simulink model "MATLABPSB_BASED_MODELING_AND_Sim"  (Simulink 8.1)
settings: Solver=FixedStepDiscrete  SolverMode=SingleTasking  StartTime=0.0  StopTime=1  FixedStep=Ts  MaxStep=Ts*2  RelTol=1e-4  AbsTol=1e-4
PreLoadFcn:
  | Ts=50e-6;
values from neighbouring files (symbols this model uses):
  A = 1.5    [LoadSimulation.m]
undefined symbols (not defined in the file or in its folder): DiscIntNeverNeededParam, find_system
libraries: powerlib x205, powerlib_extras x39
(part 4 of 5)

== system MATLABPSB_BASED_MODELING_AND_Sim/SS1/SVC Controller/Firing Unit/Firing Unit BC/BL8 ==
  Ns/c : Inport
  Alpha : Inport  Port=2  PortDimensions=1
  Sync + : Inport  Port=3  PortDimensions=1
  SqWave : Inport  Port=4  PortDimensions=1
  Alpha 90<A<181 : Constant  Value=90
  Alpha 90<A<182 : Constant  Value=360
  Alpha 90<A<183 : Constant  Value=2
  Alpha 90<A<184 : Constant  Value=2
  Alpha 90<A<185 : Constant  Value=87
  Discrete-Time Integrator : DiscreteIntegrator  ExternalReset=rising  SampleTime=Ts  LimitOutput=on  UpperSaturationLimit=100000  LowerSaturationLimit=0  ICPrevOutput=DiscIntNeverNeededParam  ICPrevScaledInput=DiscIntNeverNeededParam
  Gain2 : Gain  Gain=1/Ts  SaturateOnIntegerOverflow=on  OutDataTypeStr=Inherit: Same as input  ParamDataTypeStr=Inherit: Same as input
  Logical Operator1 : Logic  Inputs=3
  Logical Operator2 : Logic  Operator=NOT  Inputs=3
  Product : Product  Inputs=*/  SaturateOnIntegerOverflow=on  InputSameDT=on  OutDataTypeStr=Inherit: Same as first input
  Product1 : Product  Inputs=**  SaturateOnIntegerOverflow=on  InputSameDT=on  OutDataTypeStr=Inherit: Same as first input
  Product2 : Product  Inputs=*/  SaturateOnIntegerOverflow=on  InputSameDT=on  OutDataTypeStr=Inherit: Same as first input
  Relational Operator1 : RelationalOperator  Operator=<=  InputSameDT=on
  Relational Operator2 : RelationalOperator  InputSameDT=on
  Relational Operator3 : RelationalOperator  Operator=<=  InputSameDT=on
  Rounding Function1 : Rounding  Operator=round
  Rounding Function3 : Rounding  Operator=round
  Sum1 : Sum  Inputs=+-  SaturateOnIntegerOverflow=on  InputSameDT=on  OutDataTypeStr=Inherit: Same as first input
  Sum2 : Sum  Inputs=+--  SaturateOnIntegerOverflow=on  InputSameDT=on  OutDataTypeStr=Inherit: Same as first input
  Switch : Switch  Threshold=0.5  SaturateOnIntegerOverflow=on  InputSameDT=on
  Switch1 : Switch  Threshold=0.5  SaturateOnIntegerOverflow=on  InputSameDT=on
  Unit Delay1 : UnitDelay  InitialCondition=180  SampleTime=Ts
  TCR + : Outport
  wires:
  Switch1/1 -> Sum1/1, Unit Delay1/1
  Alpha 90<A<181/1 -> Sum1/2
  Ns/c/1 -> Product1/1, Product2/1
  Product1/1 -> Rounding Function1/1
  Alpha 90<A<182/1 -> Product/2
  Product/1 -> Product1/2
  Product2/1 -> Rounding Function3/1
  Alpha 90<A<183/1 -> Product2/2
  Sum1/1 -> Product/1, Relational Operator1/1
  Alpha 90<A<185/1 -> Relational Operator1/2
  Unit Delay1/1 -> Switch1/3
  Alpha/1 -> Switch1/1
  Rounding Function1/1 -> Sum2/3, Switch/1
  Rounding Function3/1 -> Sum2/1, Switch/3
  Alpha 90<A<184/1 -> Sum2/2
  Relational Operator1/1 -> Switch/2
  Relational Operator3/1 -> Logical Operator1/3
  Discrete-Time Integrator/1 -> Relational Operator2/1, Relational Operator3/1
  Relational Operator2/1 -> Logical Operator1/2
  Logical Operator1/1 -> TCR +/1
  Gain2/1 -> Discrete-Time Integrator/1
  Switch/1 -> Relational Operator2/2
  Sum2/1 -> Relational Operator3/2
  Logical Operator2/1 -> Discrete-Time Integrator/2
  Sync +/1 -> Switch1/2
  SqWave/1 -> Gain2/1, Logical Operator2/1, Logical Operator1/1

== system MATLABPSB_BASED_MODELING_AND_Sim/SS1/SVC Controller/Firing Unit/Firing Unit CA/BL1 ==
  note: Pierre Giroux, Gilbert Sybille
      | Power System Laboratory, IREQ
      | Hydro-Quebec
  note: Note: PLL synchronized on positive peak of input
  note: Discrete 1-phase PLL
  note: Note: -sin( a ) * sin( b ) = 1/2 * cos( a+b ) - 1/2 * cos(a-b)
  V(pu) : Inport
  Constant4 : Constant  Value=2*pi
  Discrete PI Controller : powerlib_extras/Discrete  Control Blocks/Discrete PI Controller  Kp=Kp  Ki=Ki  Par_Limits="[1.25  0.75]*2*pi*Finit"  Init=2*pi*Finit  Ts=Ts
  Discrete Rate Limiter : powerlib_extras/Discrete  Control Blocks/Discrete Rate Limiter  R=10  F=-10  Vinit=Finit  Ts=Ts
  Discrete Variable Frequency Mean value : powerlib_extras/Discrete Measurements/Discrete Variable Frequency Mean value  Finit=Finit  Fmin=45  Vinit=0  Ts=Ts
  Discrete  2nd-Order Filter : powerlib_extras/Discrete  Control Blocks/Discrete  2nd-Order Filter  FilterType=Lowpass  Fo=25  Zeta=0.707  Ts=Ts  Initialize=on  Vac_Init="[0 0  Finit]"  Vdc_Init=Finit  PlotResponse=off  param1=[1 500 0.1]
  Discrete-Time Integrator : DiscreteIntegrator  InitialCondition=(Phase_Init-90)*pi/180  SampleTime=Ts  ICPrevOutput=DiscIntNeverNeededParam  ICPrevScaledInput=DiscIntNeverNeededParam
  Gain10 : Gain  Gain=1/2/pi  SaturateOnIntegerOverflow=on  OutDataTypeStr=Inherit: Same as input  ParamDataTypeStr=Inherit: Same as input
  Gain12 : Gain  Gain=-1  SaturateOnIntegerOverflow=on  OutDataTypeStr=Inherit: Same as input  ParamDataTypeStr=Inherit: Same as input
  Math Function : Math  Operator=mod  SaturateOnIntegerOverflow=on
  Product1 : Product  SaturateOnIntegerOverflow=on  InputSameDT=on  OutDataTypeStr=Inherit: Same as first input
  Trigonometric Function6 : Trigonometry
  Unit Delay1 : UnitDelay  InitialCondition=Finit  SampleTime=Ts
  Freq : Outport
  wt : Outport  Port=2
  wires:
  Math Function/1 -> wt/1, Trigonometric Function6/1
  Trigonometric Function6/1 -> Product1/2
  Unit Delay1/1 -> Discrete Variable Frequency Mean value/1, Freq/1
  Discrete  2nd-Order Filter/1 -> Unit Delay1/1
  Discrete Rate Limiter/1 -> Discrete  2nd-Order Filter/1
  Gain10/1 -> Discrete Rate Limiter/1
  Discrete PI Controller/1 -> Gain10/1, Discrete-Time Integrator/1  "W"
  Product1/1 -> Discrete Variable Frequency Mean value/2
  Discrete Variable Frequency Mean value/1 -> Discrete PI Controller/1
  Discrete-Time Integrator/1 -> Math Function/1
  Constant4/1 -> Math Function/2
  V(pu)/1 -> Gain12/1
  Gain12/1 -> Product1/1

== system MATLABPSB_BASED_MODELING_AND_Sim/SS1/SVC Controller/Firing Unit/Firing Unit CA/BL2 ==
  Freq : Inport  PortDimensions=1
  Constant1 : Constant  Value=0
  Constant2 : Constant  Value=1e-5
  Constant3 : Constant
  Gain : Gain  Gain=Ts  SaturateOnIntegerOverflow=on  OutDataTypeStr=Inherit: Same as input  ParamDataTypeStr=Inherit: Same as input
  Product : Product  Inputs=/*  SaturateOnIntegerOverflow=on  InputSameDT=on  OutDataTypeStr=Inherit: Same as first input
  Relational Operator1 : RelationalOperator  Operator=~=  InputSameDT=on
  Switch : Switch  Threshold=0.5  SaturateOnIntegerOverflow=on  InputSameDT=on
  Ns/c : Outport
  wires:
  Constant3/1 -> Product/2
  Switch/1 -> Product/1
  Relational Operator1/1 -> Switch/2
  Constant2/1 -> Switch/3
  Gain/1 -> Switch/1, Relational Operator1/1
  Constant1/1 -> Relational Operator1/2
  Freq/1 -> Gain/1
  Product/1 -> Ns/c/1

== system MATLABPSB_BASED_MODELING_AND_Sim/SS1/SVC Controller/Firing Unit/Firing Unit CA/BL3 ==
  Freq : Inport  PortDimensions=1
  sin(wt) : Inport  Port=2  PortDimensions=1
  Latch : Subsystem
  Logical Operator2 : Logic
  Logical Operator4 : Logic
  Product2 : Product  SaturateOnIntegerOverflow=on  InputSameDT=on  OutDataTypeStr=Inherit: Same as first input
  Relational Operator : RelationalOperator  Operator=>  InputSameDT=on
  Relational Operator1 : RelationalOperator  Operator=>  InputSameDT=on
  Relational Operator2 : RelationalOperator  Operator=<  InputSameDT=on
  Relational Operator3 : RelationalOperator  Operator=<  InputSameDT=on
  Scope : Scope
      settings: YMin=-0.0004  YMax=0.0004  SampleInput=on  SampleTime=Ts
  Sum5 : Sum  Inputs=+-  SaturateOnIntegerOverflow=on  InputSameDT=on  OutDataTypeStr=Inherit: Same as first input
  Sum6 : Sum  SaturateOnIntegerOverflow=on  InputSameDT=on  OutDataTypeStr=Inherit: Same as first input
  Trigonometric Function7 : Trigonometry
  Unit Delay : UnitDelay  SampleTime=Ts
  Unit Delay1 : UnitDelay  SampleTime=Ts
  Unit Delay2 : UnitDelay  SampleTime=Ts
  alpha2 : Constant  Value=0
  alpha9 : Constant  Value=pi*Ts
  SqWave : Outport
  Sync + : Outport  Port=2
  Sync - : Outport  Port=3
  wires:
  alpha9/1 -> Product2/1
  Product2/1 -> Trigonometric Function7/1
  Latch/1(1) -> SqWave/1, Unit Delay1/1, Unit Delay2/1, Relational Operator1/1, Relational Operator3/1
  Unit Delay1/1 -> Logical Operator4/2
  Logical Operator4/1 -> Latch/2(R)
  Relational Operator2/1 -> Logical Operator4/1
  Unit Delay/1 -> Logical Operator2/2
  Latch/2(0) -> Unit Delay/1
  Logical Operator2/1 -> Latch/1(S)
  Relational Operator/1 -> Logical Operator2/1
  Sum6/1 -> Relational Operator2/2
  Sum5/1 -> Relational Operator/2
  alpha2/1 -> Sum6/1, Sum5/1
  Relational Operator1/1 -> Sync +/1
  Relational Operator3/1 -> Sync -/1
  Unit Delay2/1 -> Relational Operator1/2, Relational Operator3/2
  Trigonometric Function7/1 -> Sum6/2, Sum5/2, Scope/1
  Freq/1 -> Product2/2
  sin(wt)/1 -> Relational Operator/1, Relational Operator2/1

== system MATLABPSB_BASED_MODELING_AND_Sim/SS1/SVC Controller/Firing Unit/Firing Unit CA/BL4 ==
  note: Note: Sync+ , Sync - and SqWave signals are inverted for TSC firing (i.e. positive thyristor is fired on negative peak voltage)
  SqWave : Inport  PortDimensions=1
  Sync + : Inport  Port=2  PortDimensions=1
  Sync - : Inport  Port=3  PortDimensions=1
  TSC_On : Inport  Port=4  PortDimensions=1
  Alpha1 : Constant  Value=FiringMode-1
  Logical Operator1 : Logic  Operator=NOT
  Logical Operator10 : Logic  Operator=OR
  Logical Operator11 : Logic  Inputs=3
  Logical Operator12 : Logic
  Logical Operator13 : Logic
  Logical Operator14 : Logic  Operator=OR
  Logical Operator15 : Logic  Inputs=3
  Switch5 : Switch  Threshold=0.5  SaturateOnIntegerOverflow=on  InputSameDT=on
  Switch6 : Switch  Threshold=0.5  SaturateOnIntegerOverflow=on  InputSameDT=on
  Transport Delay : TransportDelay  DelayTime=1/FreqInit  BufferSize=2048
  Unit Delay6 : UnitDelay  SampleTime=Ts
  Unit Delay7 : UnitDelay  SampleTime=Ts
  TSC + : Outport
  TSC - : Outport  Port=2
  wires:
  Transport Delay/1 -> Logical Operator14/2, Logical Operator10/2
  Logical Operator15/1 -> TSC -/1
  Logical Operator11/1 -> TSC +/1
  Logical Operator14/1 -> Logical Operator15/2
  Logical Operator10/1 -> Logical Operator11/2
  Logical Operator1/1 -> Logical Operator10/1
  Switch6/1 -> Logical Operator15/1, Logical Operator13/2, Unit Delay7/1
  Switch5/1 -> Logical Operator11/1, Logical Operator13/1, Unit Delay6/1
  SqWave/1 -> Logical Operator14/1, Logical Operator1/1
  Logical Operator12/1 -> Transport Delay/1
  Alpha1/1 -> Logical Operator12/2
  Logical Operator13/1 -> Logical Operator12/1
  TSC_On/1 -> Logical Operator15/3, Logical Operator11/3, Switch6/1, Switch5/1
  Sync -/1 -> Switch5/2
  Sync +/1 -> Switch6/2
  Unit Delay7/1 -> Switch6/3
  Unit Delay6/1 -> Switch5/3

== system MATLABPSB_BASED_MODELING_AND_Sim/SS1/SVC Controller/Firing Unit/Firing Unit CA/BL5 ==
  note: Note: Sync+ , Sync - and SqWave signals are inverted for TSC firing (i.e. positive thyristor is fired on negative peak voltage)
  SqWave : Inport  PortDimensions=1
  Sync + : Inport  Port=2  PortDimensions=1
  Sync - : Inport  Port=3  PortDimensions=1
  TSC_On : Inport  Port=4  PortDimensions=1
  Alpha1 : Constant  Value=FiringMode-1
  Logical Operator1 : Logic  Operator=NOT
  Logical Operator10 : Logic  Operator=OR
  Logical Operator11 : Logic  Inputs=3
  Logical Operator12 : Logic
  Logical Operator13 : Logic
  Logical Operator14 : Logic  Operator=OR
  Logical Operator15 : Logic  Inputs=3
  Switch5 : Switch  Threshold=0.5  SaturateOnIntegerOverflow=on  InputSameDT=on
  Switch6 : Switch  Threshold=0.5  SaturateOnIntegerOverflow=on  InputSameDT=on
  Transport Delay : TransportDelay  DelayTime=1/FreqInit  BufferSize=2048
  Unit Delay6 : UnitDelay  SampleTime=Ts
  Unit Delay7 : UnitDelay  SampleTime=Ts
  TSC + : Outport
  TSC - : Outport  Port=2
  wires:
  Unit Delay6/1 -> Switch5/3
  Unit Delay7/1 -> Switch6/3
  Sync +/1 -> Switch6/2
  Sync -/1 -> Switch5/2
  TSC_On/1 -> Switch5/1, Switch6/1, Logical Operator11/3, Logical Operator15/3
  Logical Operator13/1 -> Logical Operator12/1
  Alpha1/1 -> Logical Operator12/2
  Logical Operator12/1 -> Transport Delay/1
  SqWave/1 -> Logical Operator1/1, Logical Operator14/1
  Switch5/1 -> Unit Delay6/1, Logical Operator13/1, Logical Operator11/1
  Switch6/1 -> Unit Delay7/1, Logical Operator13/2, Logical Operator15/1
  Logical Operator1/1 -> Logical Operator10/1
  Logical Operator10/1 -> Logical Operator11/2
  Logical Operator14/1 -> Logical Operator15/2
  Logical Operator11/1 -> TSC +/1
  Logical Operator15/1 -> TSC -/1
  Transport Delay/1 -> Logical Operator10/2, Logical Operator14/2

== system MATLABPSB_BASED_MODELING_AND_Sim/SS1/SVC Controller/Firing Unit/Firing Unit CA/BL6 ==
  note: Note: Sync+ , Sync - and SqWave signals are inverted for TSC firing (i.e. positive thyristor is fired on negative peak voltage)
  SqWave : Inport  PortDimensions=1
  Sync + : Inport  Port=2  PortDimensions=1
  Sync - : Inport  Port=3  PortDimensions=1
  TSC_On : Inport  Port=4  PortDimensions=1
  Alpha1 : Constant  Value=FiringMode-1
  Logical Operator1 : Logic  Operator=NOT
  Logical Operator10 : Logic  Operator=OR
  Logical Operator11 : Logic  Inputs=3
  Logical Operator12 : Logic
  Logical Operator13 : Logic
  Logical Operator14 : Logic  Operator=OR
  Logical Operator15 : Logic  Inputs=3
  Switch5 : Switch  Threshold=0.5  SaturateOnIntegerOverflow=on  InputSameDT=on
  Switch6 : Switch  Threshold=0.5  SaturateOnIntegerOverflow=on  InputSameDT=on
  Transport Delay : TransportDelay  DelayTime=1/FreqInit  BufferSize=2048
  Unit Delay6 : UnitDelay  SampleTime=Ts
  Unit Delay7 : UnitDelay  SampleTime=Ts
  TSC + : Outport
  TSC - : Outport  Port=2
  wires:
  Transport Delay/1 -> Logical Operator14/2, Logical Operator10/2
  Logical Operator15/1 -> TSC -/1
  Logical Operator11/1 -> TSC +/1
  Logical Operator14/1 -> Logical Operator15/2
  Logical Operator10/1 -> Logical Operator11/2
  Logical Operator1/1 -> Logical Operator10/1
  Switch6/1 -> Logical Operator15/1, Logical Operator13/2, Unit Delay7/1
  Switch5/1 -> Logical Operator11/1, Logical Operator13/1, Unit Delay6/1
  SqWave/1 -> Logical Operator14/1, Logical Operator1/1
  Logical Operator12/1 -> Transport Delay/1
  Alpha1/1 -> Logical Operator12/2
  Logical Operator13/1 -> Logical Operator12/1
  TSC_On/1 -> Logical Operator15/3, Logical Operator11/3, Switch6/1, Switch5/1
  Sync -/1 -> Switch5/2
  Sync +/1 -> Switch6/2
  Unit Delay7/1 -> Switch6/3
  Unit Delay6/1 -> Switch5/3

== system MATLABPSB_BASED_MODELING_AND_Sim/SS1/SVC Controller/Firing Unit/Firing Unit CA/BL7 ==
  Ns/c : Inport
  Alpha : Inport  Port=2  PortDimensions=1
  Sync - : Inport  Port=3  PortDimensions=1
  SqWave : Inport  Port=4  PortDimensions=1
  Alpha 90<A<181 : Constant  Value=90
  Alpha 90<A<182 : Constant  Value=360
  Alpha 90<A<183 : Constant  Value=2
  Alpha 90<A<184 : Constant  Value=2
  Alpha 90<A<185 : Constant  Value=87
  Discrete-Time Integrator : DiscreteIntegrator  ExternalReset=rising  SampleTime=Ts  LimitOutput=on  UpperSaturationLimit=100000  LowerSaturationLimit=0  ICPrevOutput=DiscIntNeverNeededParam  ICPrevScaledInput=DiscIntNeverNeededParam
  Gain2 : Gain  Gain=1/Ts  SaturateOnIntegerOverflow=on  OutDataTypeStr=Inherit: Same as input  ParamDataTypeStr=Inherit: Same as input
  Logical Operator1 : Logic  Inputs=3
  Logical Operator2 : Logic  Operator=NOT  Inputs=3
  Logical Operator3 : Logic  Operator=NOT  Inputs=3
  Product : Product  Inputs=*/  SaturateOnIntegerOverflow=on  InputSameDT=on  OutDataTypeStr=Inherit: Same as first input
  Product1 : Product  Inputs=**  SaturateOnIntegerOverflow=on  InputSameDT=on  OutDataTypeStr=Inherit: Same as first input
  Product2 : Product  Inputs=*/  SaturateOnIntegerOverflow=on  InputSameDT=on  OutDataTypeStr=Inherit: Same as first input
  Relational Operator1 : RelationalOperator  Operator=<=  InputSameDT=on
  Relational Operator2 : RelationalOperator  InputSameDT=on
  Relational Operator3 : RelationalOperator  Operator=<=  InputSameDT=on
  Rounding Function1 : Rounding  Operator=round
  Rounding Function3 : Rounding  Operator=round
  Sum1 : Sum  Inputs=+-  SaturateOnIntegerOverflow=on  InputSameDT=on  OutDataTypeStr=Inherit: Same as first input
  Sum2 : Sum  Inputs=+--  SaturateOnIntegerOverflow=on  InputSameDT=on  OutDataTypeStr=Inherit: Same as first input
  Switch : Switch  Threshold=0.5  SaturateOnIntegerOverflow=on  InputSameDT=on
  Switch1 : Switch  Threshold=0.5  SaturateOnIntegerOverflow=on  InputSameDT=on
  Unit Delay1 : UnitDelay  InitialCondition=180  SampleTime=Ts
  TCR - : Outport
  wires:
  Switch1/1 -> Sum1/1, Unit Delay1/1
  Alpha 90<A<181/1 -> Sum1/2
  Ns/c/1 -> Product1/1, Product2/1
  Product1/1 -> Rounding Function1/1
  Alpha 90<A<182/1 -> Product/2
  Product/1 -> Product1/2
  Product2/1 -> Rounding Function3/1
  Alpha 90<A<183/1 -> Product2/2
  Sum1/1 -> Product/1, Relational Operator1/1
  Alpha 90<A<185/1 -> Relational Operator1/2
  Unit Delay1/1 -> Switch1/3
  Alpha/1 -> Switch1/1
  Rounding Function1/1 -> Sum2/3, Switch/1
  Rounding Function3/1 -> Sum2/1, Switch/3
  Alpha 90<A<184/1 -> Sum2/2
  Relational Operator1/1 -> Switch/2
  Relational Operator3/1 -> Logical Operator1/3
  Discrete-Time Integrator/1 -> Relational Operator2/1, Relational Operator3/1
  Relational Operator2/1 -> Logical Operator1/2
  Logical Operator1/1 -> TCR -/1
  Gain2/1 -> Discrete-Time Integrator/1
  Switch/1 -> Relational Operator2/2
  Sum2/1 -> Relational Operator3/2
  Logical Operator2/1 -> Discrete-Time Integrator/2
  Sync -/1 -> Switch1/2
  SqWave/1 -> Logical Operator3/1
  Logical Operator3/1 -> Gain2/1, Logical Operator2/1, Logical Operator1/1

== system MATLABPSB_BASED_MODELING_AND_Sim/SS1/SVC Controller/Firing Unit/Firing Unit CA/BL8 ==
  Ns/c : Inport
  Alpha : Inport  Port=2  PortDimensions=1
  Sync + : Inport  Port=3  PortDimensions=1
  SqWave : Inport  Port=4  PortDimensions=1
  Alpha 90<A<181 : Constant  Value=90
  Alpha 90<A<182 : Constant  Value=360
  Alpha 90<A<183 : Constant  Value=2
  Alpha 90<A<184 : Constant  Value=2
  Alpha 90<A<185 : Constant  Value=87
  Discrete-Time Integrator : DiscreteIntegrator  ExternalReset=rising  SampleTime=Ts  LimitOutput=on  UpperSaturationLimit=100000  LowerSaturationLimit=0  ICPrevOutput=DiscIntNeverNeededParam  ICPrevScaledInput=DiscIntNeverNeededParam
  Gain2 : Gain  Gain=1/Ts  SaturateOnIntegerOverflow=on  OutDataTypeStr=Inherit: Same as input  ParamDataTypeStr=Inherit: Same as input
  Logical Operator1 : Logic  Inputs=3
  Logical Operator2 : Logic  Operator=NOT  Inputs=3
  Product : Product  Inputs=*/  SaturateOnIntegerOverflow=on  InputSameDT=on  OutDataTypeStr=Inherit: Same as first input
  Product1 : Product  Inputs=**  SaturateOnIntegerOverflow=on  InputSameDT=on  OutDataTypeStr=Inherit: Same as first input
  Product2 : Product  Inputs=*/  SaturateOnIntegerOverflow=on  InputSameDT=on  OutDataTypeStr=Inherit: Same as first input
  Relational Operator1 : RelationalOperator  Operator=<=  InputSameDT=on
  Relational Operator2 : RelationalOperator  InputSameDT=on
  Relational Operator3 : RelationalOperator  Operator=<=  InputSameDT=on
  Rounding Function1 : Rounding  Operator=round
  Rounding Function3 : Rounding  Operator=round
  Sum1 : Sum  Inputs=+-  SaturateOnIntegerOverflow=on  InputSameDT=on  OutDataTypeStr=Inherit: Same as first input
  Sum2 : Sum  Inputs=+--  SaturateOnIntegerOverflow=on  InputSameDT=on  OutDataTypeStr=Inherit: Same as first input
  Switch : Switch  Threshold=0.5  SaturateOnIntegerOverflow=on  InputSameDT=on
  Switch1 : Switch  Threshold=0.5  SaturateOnIntegerOverflow=on  InputSameDT=on
  Unit Delay1 : UnitDelay  InitialCondition=180  SampleTime=Ts
  TCR + : Outport
  wires:
  SqWave/1 -> Logical Operator1/1, Logical Operator2/1, Gain2/1
  Sync +/1 -> Switch1/2
  Logical Operator2/1 -> Discrete-Time Integrator/2
  Sum2/1 -> Relational Operator3/2
  Switch/1 -> Relational Operator2/2
  Gain2/1 -> Discrete-Time Integrator/1
  Logical Operator1/1 -> TCR +/1
  Relational Operator2/1 -> Logical Operator1/2
  Discrete-Time Integrator/1 -> Relational Operator3/1, Relational Operator2/1
  Relational Operator3/1 -> Logical Operator1/3
  Relational Operator1/1 -> Switch/2
  Alpha 90<A<184/1 -> Sum2/2
  Rounding Function3/1 -> Switch/3, Sum2/1
  Rounding Function1/1 -> Switch/1, Sum2/3
  Alpha/1 -> Switch1/1
  Unit Delay1/1 -> Switch1/3
  Alpha 90<A<185/1 -> Relational Operator1/2
  Sum1/1 -> Relational Operator1/1, Product/1
  Alpha 90<A<183/1 -> Product2/2
  Product2/1 -> Rounding Function3/1
  Product/1 -> Product1/2
  Alpha 90<A<182/1 -> Product/2
  Product1/1 -> Rounding Function1/1
  Ns/c/1 -> Product2/1, Product1/1
  Alpha 90<A<181/1 -> Sum1/2
  Switch1/1 -> Unit Delay1/1, Sum1/1

== system MATLABPSB_BASED_MODELING_AND_Sim/SS2/SVC Controller/Firing Unit/Firing Unit AB/BL1 ==
  note: Pierre Giroux, Gilbert Sybille
      | Power System Laboratory, IREQ
      | Hydro-Quebec
  note: Note: PLL synchronized on positive peak of input
  note: Discrete 1-phase PLL
  note: Note: -sin( a ) * sin( b ) = 1/2 * cos( a+b ) - 1/2 * cos(a-b)
  V(pu) : Inport
  Constant4 : Constant  Value=2*pi
  Discrete PI Controller : powerlib_extras/Discrete  Control Blocks/Discrete PI Controller  Kp=Kp  Ki=Ki  Par_Limits="[1.25  0.75]*2*pi*Finit"  Init=2*pi*Finit  Ts=Ts
  Discrete Rate Limiter : powerlib_extras/Discrete  Control Blocks/Discrete Rate Limiter  R=10  F=-10  Vinit=Finit  Ts=Ts
  Discrete Variable Frequency Mean value : powerlib_extras/Discrete Measurements/Discrete Variable Frequency Mean value  Finit=Finit  Fmin=45  Vinit=0  Ts=Ts
  Discrete  2nd-Order Filter : powerlib_extras/Discrete  Control Blocks/Discrete  2nd-Order Filter  FilterType=Lowpass  Fo=25  Zeta=0.707  Ts=Ts  Initialize=on  Vac_Init="[0 0  Finit]"  Vdc_Init=Finit  PlotResponse=off  param1=[1 500 0.1]
  Discrete-Time Integrator : DiscreteIntegrator  InitialCondition=(Phase_Init-90)*pi/180  SampleTime=Ts  ICPrevOutput=DiscIntNeverNeededParam  ICPrevScaledInput=DiscIntNeverNeededParam
  Gain10 : Gain  Gain=1/2/pi  SaturateOnIntegerOverflow=on  OutDataTypeStr=Inherit: Same as input  ParamDataTypeStr=Inherit: Same as input
  Gain12 : Gain  Gain=-1  SaturateOnIntegerOverflow=on  OutDataTypeStr=Inherit: Same as input  ParamDataTypeStr=Inherit: Same as input
  Math Function : Math  Operator=mod  SaturateOnIntegerOverflow=on
  Product1 : Product  SaturateOnIntegerOverflow=on  InputSameDT=on  OutDataTypeStr=Inherit: Same as first input
  Trigonometric Function6 : Trigonometry
  Unit Delay1 : UnitDelay  InitialCondition=Finit  SampleTime=Ts
  Freq : Outport
  wt : Outport  Port=2
  wires:
  Math Function/1 -> wt/1, Trigonometric Function6/1
  Trigonometric Function6/1 -> Product1/2
  Unit Delay1/1 -> Discrete Variable Frequency Mean value/1, Freq/1
  Discrete  2nd-Order Filter/1 -> Unit Delay1/1
  Discrete Rate Limiter/1 -> Discrete  2nd-Order Filter/1
  Gain10/1 -> Discrete Rate Limiter/1
  Discrete PI Controller/1 -> Gain10/1, Discrete-Time Integrator/1  "W"
  Product1/1 -> Discrete Variable Frequency Mean value/2
  Discrete Variable Frequency Mean value/1 -> Discrete PI Controller/1
  Discrete-Time Integrator/1 -> Math Function/1
  Constant4/1 -> Math Function/2
  V(pu)/1 -> Gain12/1
  Gain12/1 -> Product1/1

== system MATLABPSB_BASED_MODELING_AND_Sim/SS2/SVC Controller/Firing Unit/Firing Unit AB/BL2 ==
  Freq : Inport  PortDimensions=1
  Constant1 : Constant  Value=0
  Constant2 : Constant  Value=1e-5
  Constant3 : Constant
  Gain : Gain  Gain=Ts  SaturateOnIntegerOverflow=on  OutDataTypeStr=Inherit: Same as input  ParamDataTypeStr=Inherit: Same as input
  Product : Product  Inputs=/*  SaturateOnIntegerOverflow=on  InputSameDT=on  OutDataTypeStr=Inherit: Same as first input
  Relational Operator1 : RelationalOperator  Operator=~=  InputSameDT=on
  Switch : Switch  Threshold=0.5  SaturateOnIntegerOverflow=on  InputSameDT=on
  Ns/c : Outport
  wires:
  Constant3/1 -> Product/2
  Switch/1 -> Product/1
  Relational Operator1/1 -> Switch/2
  Constant2/1 -> Switch/3
  Gain/1 -> Switch/1, Relational Operator1/1
  Constant1/1 -> Relational Operator1/2
  Freq/1 -> Gain/1
  Product/1 -> Ns/c/1

== system MATLABPSB_BASED_MODELING_AND_Sim/SS2/SVC Controller/Firing Unit/Firing Unit AB/BL3 ==
  Freq : Inport  PortDimensions=1
  sin(wt) : Inport  Port=2  PortDimensions=1
  Latch : Subsystem
  Logical Operator2 : Logic
  Logical Operator4 : Logic
  Product2 : Product  SaturateOnIntegerOverflow=on  InputSameDT=on  OutDataTypeStr=Inherit: Same as first input
  Relational Operator : RelationalOperator  Operator=>  InputSameDT=on
  Relational Operator1 : RelationalOperator  Operator=>  InputSameDT=on
  Relational Operator2 : RelationalOperator  Operator=<  InputSameDT=on
  Relational Operator3 : RelationalOperator  Operator=<  InputSameDT=on
  Scope : Scope
      settings: YMin=-0.0004  YMax=0.0004  SampleInput=on  SampleTime=Ts
  Sum5 : Sum  Inputs=+-  SaturateOnIntegerOverflow=on  InputSameDT=on  OutDataTypeStr=Inherit: Same as first input
  Sum6 : Sum  SaturateOnIntegerOverflow=on  InputSameDT=on  OutDataTypeStr=Inherit: Same as first input
  Trigonometric Function7 : Trigonometry
  Unit Delay : UnitDelay  SampleTime=Ts
  Unit Delay1 : UnitDelay  SampleTime=Ts
  Unit Delay2 : UnitDelay  SampleTime=Ts
  alpha2 : Constant  Value=0
  alpha9 : Constant  Value=pi*Ts
  SqWave : Outport
  Sync + : Outport  Port=2
  Sync - : Outport  Port=3
  wires:
  alpha9/1 -> Product2/1
  Product2/1 -> Trigonometric Function7/1
  Latch/1(1) -> SqWave/1, Unit Delay1/1, Unit Delay2/1, Relational Operator1/1, Relational Operator3/1
  Unit Delay1/1 -> Logical Operator4/2
  Logical Operator4/1 -> Latch/2(R)
  Relational Operator2/1 -> Logical Operator4/1
  Unit Delay/1 -> Logical Operator2/2
  Latch/2(0) -> Unit Delay/1
  Logical Operator2/1 -> Latch/1(S)
  Relational Operator/1 -> Logical Operator2/1
  Sum6/1 -> Relational Operator2/2
  Sum5/1 -> Relational Operator/2
  alpha2/1 -> Sum6/1, Sum5/1
  Relational Operator1/1 -> Sync +/1
  Relational Operator3/1 -> Sync -/1
  Unit Delay2/1 -> Relational Operator1/2, Relational Operator3/2
  Trigonometric Function7/1 -> Scope/1, Sum6/2, Sum5/2
  Freq/1 -> Product2/2
  sin(wt)/1 -> Relational Operator/1, Relational Operator2/1

== system MATLABPSB_BASED_MODELING_AND_Sim/SS2/SVC Controller/Firing Unit/Firing Unit AB/BL4 ==
  Ns/c : Inport
  Alpha : Inport  Port=2  PortDimensions=1
  Sync + : Inport  Port=3  PortDimensions=1
  SqWave : Inport  Port=4  PortDimensions=1
  Alpha 90<A<181 : Constant  Value=90
  Alpha 90<A<182 : Constant  Value=360
  Alpha 90<A<183 : Constant  Value=2
  Alpha 90<A<184 : Constant  Value=2
  Alpha 90<A<185 : Constant  Value=87
  Discrete-Time Integrator : DiscreteIntegrator  ExternalReset=rising  SampleTime=Ts  LimitOutput=on  UpperSaturationLimit=100000  LowerSaturationLimit=0  ICPrevOutput=DiscIntNeverNeededParam  ICPrevScaledInput=DiscIntNeverNeededParam
  Gain2 : Gain  Gain=1/Ts  SaturateOnIntegerOverflow=on  OutDataTypeStr=Inherit: Same as input  ParamDataTypeStr=Inherit: Same as input
  Logical Operator1 : Logic  Inputs=3
  Logical Operator2 : Logic  Operator=NOT  Inputs=3
  Product : Product  Inputs=*/  SaturateOnIntegerOverflow=on  InputSameDT=on  OutDataTypeStr=Inherit: Same as first input
  Product1 : Product  Inputs=**  SaturateOnIntegerOverflow=on  InputSameDT=on  OutDataTypeStr=Inherit: Same as first input
  Product2 : Product  Inputs=*/  SaturateOnIntegerOverflow=on  InputSameDT=on  OutDataTypeStr=Inherit: Same as first input
  Relational Operator1 : RelationalOperator  Operator=<=  InputSameDT=on
  Relational Operator2 : RelationalOperator  InputSameDT=on
  Relational Operator3 : RelationalOperator  Operator=<=  InputSameDT=on
  Rounding Function1 : Rounding  Operator=round
  Rounding Function3 : Rounding  Operator=round
  Sum1 : Sum  Inputs=+-  SaturateOnIntegerOverflow=on  InputSameDT=on  OutDataTypeStr=Inherit: Same as first input
  Sum2 : Sum  Inputs=+--  SaturateOnIntegerOverflow=on  InputSameDT=on  OutDataTypeStr=Inherit: Same as first input
  Switch : Switch  Threshold=0.5  SaturateOnIntegerOverflow=on  InputSameDT=on
  Switch1 : Switch  Threshold=0.5  SaturateOnIntegerOverflow=on  InputSameDT=on
  Unit Delay1 : UnitDelay  InitialCondition=180  SampleTime=Ts
  TCR + : Outport
  wires:
  SqWave/1 -> Logical Operator1/1, Logical Operator2/1, Gain2/1
  Sync +/1 -> Switch1/2
  Logical Operator2/1 -> Discrete-Time Integrator/2
  Sum2/1 -> Relational Operator3/2
  Switch/1 -> Relational Operator2/2
  Gain2/1 -> Discrete-Time Integrator/1
  Logical Operator1/1 -> TCR +/1
  Relational Operator2/1 -> Logical Operator1/2
  Discrete-Time Integrator/1 -> Relational Operator3/1, Relational Operator2/1
  Relational Operator3/1 -> Logical Operator1/3
  Relational Operator1/1 -> Switch/2
  Alpha 90<A<184/1 -> Sum2/2
  Rounding Function3/1 -> Switch/3, Sum2/1
  Rounding Function1/1 -> Switch/1, Sum2/3
  Alpha/1 -> Switch1/1
  Unit Delay1/1 -> Switch1/3
  Alpha 90<A<185/1 -> Relational Operator1/2
  Sum1/1 -> Relational Operator1/1, Product/1
  Alpha 90<A<183/1 -> Product2/2
  Product2/1 -> Rounding Function3/1
  Product/1 -> Product1/2
  Alpha 90<A<182/1 -> Product/2
  Product1/1 -> Rounding Function1/1
  Ns/c/1 -> Product2/1, Product1/1
  Alpha 90<A<181/1 -> Sum1/2
  Switch1/1 -> Unit Delay1/1, Sum1/1

== system MATLABPSB_BASED_MODELING_AND_Sim/SS2/SVC Controller/Firing Unit/Firing Unit AB/BL5 ==
  Ns/c : Inport
  Alpha : Inport  Port=2  PortDimensions=1
  Sync - : Inport  Port=3  PortDimensions=1
  SqWave : Inport  Port=4  PortDimensions=1
  Alpha 90<A<181 : Constant  Value=90
  Alpha 90<A<182 : Constant  Value=360
  Alpha 90<A<183 : Constant  Value=2
  Alpha 90<A<184 : Constant  Value=2
  Alpha 90<A<185 : Constant  Value=87
  Discrete-Time Integrator : DiscreteIntegrator  ExternalReset=rising  SampleTime=Ts  LimitOutput=on  UpperSaturationLimit=100000  LowerSaturationLimit=0  ICPrevOutput=DiscIntNeverNeededParam  ICPrevScaledInput=DiscIntNeverNeededParam
  Gain2 : Gain  Gain=1/Ts  SaturateOnIntegerOverflow=on  OutDataTypeStr=Inherit: Same as input  ParamDataTypeStr=Inherit: Same as input
  Logical Operator1 : Logic  Inputs=3
  Logical Operator2 : Logic  Operator=NOT  Inputs=3
  Logical Operator3 : Logic  Operator=NOT  Inputs=3
  Product : Product  Inputs=*/  SaturateOnIntegerOverflow=on  InputSameDT=on  OutDataTypeStr=Inherit: Same as first input
  Product1 : Product  Inputs=**  SaturateOnIntegerOverflow=on  InputSameDT=on  OutDataTypeStr=Inherit: Same as first input
  Product2 : Product  Inputs=*/  SaturateOnIntegerOverflow=on  InputSameDT=on  OutDataTypeStr=Inherit: Same as first input
  Relational Operator1 : RelationalOperator  Operator=<=  InputSameDT=on
  Relational Operator2 : RelationalOperator  InputSameDT=on
  Relational Operator3 : RelationalOperator  Operator=<=  InputSameDT=on
  Rounding Function1 : Rounding  Operator=round
  Rounding Function3 : Rounding  Operator=round
  Sum1 : Sum  Inputs=+-  SaturateOnIntegerOverflow=on  InputSameDT=on  OutDataTypeStr=Inherit: Same as first input
  Sum2 : Sum  Inputs=+--  SaturateOnIntegerOverflow=on  InputSameDT=on  OutDataTypeStr=Inherit: Same as first input
  Switch : Switch  Threshold=0.5  SaturateOnIntegerOverflow=on  InputSameDT=on
  Switch1 : Switch  Threshold=0.5  SaturateOnIntegerOverflow=on  InputSameDT=on
  Unit Delay1 : UnitDelay  InitialCondition=180  SampleTime=Ts
  TCR - : Outport
  wires:
  Switch1/1 -> Sum1/1, Unit Delay1/1
  Alpha 90<A<181/1 -> Sum1/2
  Ns/c/1 -> Product1/1, Product2/1
  Product1/1 -> Rounding Function1/1
  Alpha 90<A<182/1 -> Product/2
  Product/1 -> Product1/2
  Product2/1 -> Rounding Function3/1
  Alpha 90<A<183/1 -> Product2/2
  Sum1/1 -> Product/1, Relational Operator1/1
  Alpha 90<A<185/1 -> Relational Operator1/2
  Unit Delay1/1 -> Switch1/3
  Alpha/1 -> Switch1/1
  Rounding Function1/1 -> Sum2/3, Switch/1
  Rounding Function3/1 -> Sum2/1, Switch/3
  Alpha 90<A<184/1 -> Sum2/2
  Relational Operator1/1 -> Switch/2
  Relational Operator3/1 -> Logical Operator1/3
  Discrete-Time Integrator/1 -> Relational Operator2/1, Relational Operator3/1
  Relational Operator2/1 -> Logical Operator1/2
  Logical Operator1/1 -> TCR -/1
  Gain2/1 -> Discrete-Time Integrator/1
  Switch/1 -> Relational Operator2/2
  Sum2/1 -> Relational Operator3/2
  Logical Operator2/1 -> Discrete-Time Integrator/2
  Sync -/1 -> Switch1/2
  SqWave/1 -> Logical Operator3/1
  Logical Operator3/1 -> Gain2/1, Logical Operator2/1, Logical Operator1/1

== system MATLABPSB_BASED_MODELING_AND_Sim/SS2/SVC Controller/Firing Unit/Firing Unit AB/BL6 ==
  note: Note: Sync+ , Sync - and SqWave signals are inverted for TSC firing (i.e. positive thyristor is fired on negative peak voltage)
  SqWave : Inport  PortDimensions=1
  Sync + : Inport  Port=2  PortDimensions=1
  Sync - : Inport  Port=3  PortDimensions=1
  TSC_On : Inport  Port=4  PortDimensions=1
  Alpha1 : Constant  Value=FiringMode-1
  Logical Operator1 : Logic  Operator=NOT
  Logical Operator10 : Logic  Operator=OR
  Logical Operator11 : Logic  Inputs=3
  Logical Operator12 : Logic
  Logical Operator13 : Logic
  Logical Operator14 : Logic  Operator=OR
  Logical Operator15 : Logic  Inputs=3
  Switch5 : Switch  Threshold=0.5  SaturateOnIntegerOverflow=on  InputSameDT=on
  Switch6 : Switch  Threshold=0.5  SaturateOnIntegerOverflow=on  InputSameDT=on
  Transport Delay : TransportDelay  DelayTime=1/FreqInit  BufferSize=2048
  Unit Delay6 : UnitDelay  SampleTime=Ts
  Unit Delay7 : UnitDelay  SampleTime=Ts
  TSC + : Outport
  TSC - : Outport  Port=2
  wires:
  Unit Delay6/1 -> Switch5/3
  Unit Delay7/1 -> Switch6/3
  Sync +/1 -> Switch6/2
  Sync -/1 -> Switch5/2
  TSC_On/1 -> Switch5/1, Switch6/1, Logical Operator11/3, Logical Operator15/3
  Logical Operator13/1 -> Logical Operator12/1
  Alpha1/1 -> Logical Operator12/2
  Logical Operator12/1 -> Transport Delay/1
  SqWave/1 -> Logical Operator1/1, Logical Operator14/1
  Switch5/1 -> Unit Delay6/1, Logical Operator13/1, Logical Operator11/1
  Switch6/1 -> Unit Delay7/1, Logical Operator13/2, Logical Operator15/1
  Logical Operator1/1 -> Logical Operator10/1
  Logical Operator10/1 -> Logical Operator11/2
  Logical Operator14/1 -> Logical Operator15/2
  Logical Operator11/1 -> TSC +/1
  Logical Operator15/1 -> TSC -/1
  Transport Delay/1 -> Logical Operator10/2, Logical Operator14/2

== system MATLABPSB_BASED_MODELING_AND_Sim/SS2/SVC Controller/Firing Unit/Firing Unit AB/BL7 ==
  note: Note: Sync+ , Sync - and SqWave signals are inverted for TSC firing (i.e. positive thyristor is fired on negative peak voltage)
  SqWave : Inport  PortDimensions=1
  Sync + : Inport  Port=2  PortDimensions=1
  Sync - : Inport  Port=3  PortDimensions=1
  TSC_On : Inport  Port=4  PortDimensions=1
  Alpha1 : Constant  Value=FiringMode-1
  Logical Operator1 : Logic  Operator=NOT
  Logical Operator10 : Logic  Operator=OR
  Logical Operator11 : Logic  Inputs=3
  Logical Operator12 : Logic
  Logical Operator13 : Logic
  Logical Operator14 : Logic  Operator=OR
  Logical Operator15 : Logic  Inputs=3
  Switch5 : Switch  Threshold=0.5  SaturateOnIntegerOverflow=on  InputSameDT=on
  Switch6 : Switch  Threshold=0.5  SaturateOnIntegerOverflow=on  InputSameDT=on
  Transport Delay : TransportDelay  DelayTime=1/FreqInit  BufferSize=2048
  Unit Delay6 : UnitDelay  SampleTime=Ts
  Unit Delay7 : UnitDelay  SampleTime=Ts
  TSC + : Outport
  TSC - : Outport  Port=2
  wires:
  Transport Delay/1 -> Logical Operator14/2, Logical Operator10/2
  Logical Operator15/1 -> TSC -/1
  Logical Operator11/1 -> TSC +/1
  Logical Operator14/1 -> Logical Operator15/2
  Logical Operator10/1 -> Logical Operator11/2
  Logical Operator1/1 -> Logical Operator10/1
  Switch6/1 -> Logical Operator15/1, Logical Operator13/2, Unit Delay7/1
  Switch5/1 -> Logical Operator11/1, Logical Operator13/1, Unit Delay6/1
  SqWave/1 -> Logical Operator14/1, Logical Operator1/1
  Logical Operator12/1 -> Transport Delay/1
  Alpha1/1 -> Logical Operator12/2
  Logical Operator13/1 -> Logical Operator12/1
  TSC_On/1 -> Logical Operator15/3, Logical Operator11/3, Switch6/1, Switch5/1
  Sync -/1 -> Switch5/2
  Sync +/1 -> Switch6/2
  Unit Delay7/1 -> Switch6/3
  Unit Delay6/1 -> Switch5/3

== system MATLABPSB_BASED_MODELING_AND_Sim/SS2/SVC Controller/Firing Unit/Firing Unit AB/BL8 ==
  note: Note: Sync+ , Sync - and SqWave signals are inverted for TSC firing (i.e. positive thyristor is fired on negative peak voltage)
  SqWave : Inport  PortDimensions=1
  Sync + : Inport  Port=2  PortDimensions=1
  Sync - : Inport  Port=3  PortDimensions=1
  TSC_On : Inport  Port=4  PortDimensions=1
  Alpha1 : Constant  Value=FiringMode-1
  Logical Operator1 : Logic  Operator=NOT
  Logical Operator10 : Logic  Operator=OR
  Logical Operator11 : Logic  Inputs=3
  Logical Operator12 : Logic
  Logical Operator13 : Logic
  Logical Operator14 : Logic  Operator=OR
  Logical Operator15 : Logic  Inputs=3
  Switch5 : Switch  Threshold=0.5  SaturateOnIntegerOverflow=on  InputSameDT=on
  Switch6 : Switch  Threshold=0.5  SaturateOnIntegerOverflow=on  InputSameDT=on
  Transport Delay : TransportDelay  DelayTime=1/FreqInit  BufferSize=2048
  Unit Delay6 : UnitDelay  SampleTime=Ts
  Unit Delay7 : UnitDelay  SampleTime=Ts
  TSC + : Outport
  TSC - : Outport  Port=2
  wires:
  Transport Delay/1 -> Logical Operator14/2, Logical Operator10/2
  Logical Operator15/1 -> TSC -/1
  Logical Operator11/1 -> TSC +/1
  Logical Operator14/1 -> Logical Operator15/2
  Logical Operator10/1 -> Logical Operator11/2
  Logical Operator1/1 -> Logical Operator10/1
  Switch6/1 -> Logical Operator15/1, Logical Operator13/2, Unit Delay7/1
  Switch5/1 -> Logical Operator11/1, Logical Operator13/1, Unit Delay6/1
  SqWave/1 -> Logical Operator14/1, Logical Operator1/1
  Logical Operator12/1 -> Transport Delay/1
  Alpha1/1 -> Logical Operator12/2
  Logical Operator13/1 -> Logical Operator12/1
  TSC_On/1 -> Logical Operator15/3, Logical Operator11/3, Switch6/1, Switch5/1
  Sync -/1 -> Switch5/2
  Sync +/1 -> Switch6/2
  Unit Delay7/1 -> Switch6/3
  Unit Delay6/1 -> Switch5/3

== system MATLABPSB_BASED_MODELING_AND_Sim/SS2/SVC Controller/Firing Unit/Firing Unit BC/BL1 ==
  note: Note: -sin( a ) * sin( b ) = 1/2 * cos( a+b ) - 1/2 * cos(a-b)
  note: Discrete 1-phase PLL
  note: Note: PLL synchronized on positive peak of input
  note: Pierre Giroux, Gilbert Sybille
      | Power System Laboratory, IREQ
      | Hydro-Quebec
  V(pu) : Inport
  Constant4 : Constant  Value=2*pi
  Discrete PI Controller : powerlib_extras/Discrete  Control Blocks/Discrete PI Controller  Kp=Kp  Ki=Ki  Par_Limits="[1.25  0.75]*2*pi*Finit"  Init=2*pi*Finit  Ts=Ts
  Discrete Rate Limiter : powerlib_extras/Discrete  Control Blocks/Discrete Rate Limiter  R=10  F=-10  Vinit=Finit  Ts=Ts
  Discrete Variable Frequency Mean value : powerlib_extras/Discrete Measurements/Discrete Variable Frequency Mean value  Finit=Finit  Fmin=45  Vinit=0  Ts=Ts
  Discrete  2nd-Order Filter : powerlib_extras/Discrete  Control Blocks/Discrete  2nd-Order Filter  FilterType=Lowpass  Fo=25  Zeta=0.707  Ts=Ts  Initialize=on  Vac_Init="[0 0  Finit]"  Vdc_Init=Finit  PlotResponse=off  param1=[1 500 0.1]
  Discrete-Time Integrator : DiscreteIntegrator  InitialCondition=(Phase_Init-90)*pi/180  SampleTime=Ts  ICPrevOutput=DiscIntNeverNeededParam  ICPrevScaledInput=DiscIntNeverNeededParam
  Gain10 : Gain  Gain=1/2/pi  SaturateOnIntegerOverflow=on  OutDataTypeStr=Inherit: Same as input  ParamDataTypeStr=Inherit: Same as input
  Gain12 : Gain  Gain=-1  SaturateOnIntegerOverflow=on  OutDataTypeStr=Inherit: Same as input  ParamDataTypeStr=Inherit: Same as input
  Math Function : Math  Operator=mod  SaturateOnIntegerOverflow=on
  Product1 : Product  SaturateOnIntegerOverflow=on  InputSameDT=on  OutDataTypeStr=Inherit: Same as first input
  Trigonometric Function6 : Trigonometry
  Unit Delay1 : UnitDelay  InitialCondition=Finit  SampleTime=Ts
  Freq : Outport
  wt : Outport  Port=2
  wires:
  Gain12/1 -> Product1/1
  V(pu)/1 -> Gain12/1
  Constant4/1 -> Math Function/2
  Discrete-Time Integrator/1 -> Math Function/1
  Discrete Variable Frequency Mean value/1 -> Discrete PI Controller/1
  Product1/1 -> Discrete Variable Frequency Mean value/2
  Discrete PI Controller/1 -> Discrete-Time Integrator/1, Gain10/1  "W"
  Gain10/1 -> Discrete Rate Limiter/1
  Discrete Rate Limiter/1 -> Discrete  2nd-Order Filter/1
  Discrete  2nd-Order Filter/1 -> Unit Delay1/1
  Unit Delay1/1 -> Freq/1, Discrete Variable Frequency Mean value/1
  Trigonometric Function6/1 -> Product1/2
  Math Function/1 -> Trigonometric Function6/1, wt/1

== system MATLABPSB_BASED_MODELING_AND_Sim/SS2/SVC Controller/Firing Unit/Firing Unit BC/BL2 ==
  Freq : Inport  PortDimensions=1
  Constant1 : Constant  Value=0
  Constant2 : Constant  Value=1e-5
  Constant3 : Constant
  Gain : Gain  Gain=Ts  SaturateOnIntegerOverflow=on  OutDataTypeStr=Inherit: Same as input  ParamDataTypeStr=Inherit: Same as input
  Product : Product  Inputs=/*  SaturateOnIntegerOverflow=on  InputSameDT=on  OutDataTypeStr=Inherit: Same as first input
  Relational Operator1 : RelationalOperator  Operator=~=  InputSameDT=on
  Switch : Switch  Threshold=0.5  SaturateOnIntegerOverflow=on  InputSameDT=on
  Ns/c : Outport
  wires:
  Product/1 -> Ns/c/1
  Freq/1 -> Gain/1
  Constant1/1 -> Relational Operator1/2
  Gain/1 -> Relational Operator1/1, Switch/1
  Constant2/1 -> Switch/3
  Relational Operator1/1 -> Switch/2
  Switch/1 -> Product/1
  Constant3/1 -> Product/2

== system MATLABPSB_BASED_MODELING_AND_Sim/SS2/SVC Controller/Firing Unit/Firing Unit BC/BL3 ==
  Freq : Inport  PortDimensions=1
  sin(wt) : Inport  Port=2  PortDimensions=1
  Latch : Subsystem
  Logical Operator2 : Logic
  Logical Operator4 : Logic
  Product2 : Product  SaturateOnIntegerOverflow=on  InputSameDT=on  OutDataTypeStr=Inherit: Same as first input
  Relational Operator : RelationalOperator  Operator=>  InputSameDT=on
  Relational Operator1 : RelationalOperator  Operator=>  InputSameDT=on
  Relational Operator2 : RelationalOperator  Operator=<  InputSameDT=on
  Relational Operator3 : RelationalOperator  Operator=<  InputSameDT=on
  Scope : Scope
      settings: YMin=-0.0004  YMax=0.0004  SampleInput=on  SampleTime=Ts
  Sum5 : Sum  Inputs=+-  SaturateOnIntegerOverflow=on  InputSameDT=on  OutDataTypeStr=Inherit: Same as first input
  Sum6 : Sum  SaturateOnIntegerOverflow=on  InputSameDT=on  OutDataTypeStr=Inherit: Same as first input
  Trigonometric Function7 : Trigonometry
  Unit Delay : UnitDelay  SampleTime=Ts
  Unit Delay1 : UnitDelay  SampleTime=Ts
  Unit Delay2 : UnitDelay  SampleTime=Ts
  alpha2 : Constant  Value=0
  alpha9 : Constant  Value=pi*Ts
  SqWave : Outport
  Sync + : Outport  Port=2
  Sync - : Outport  Port=3
  wires:
  sin(wt)/1 -> Relational Operator2/1, Relational Operator/1
  Freq/1 -> Product2/2
  Trigonometric Function7/1 -> Scope/1, Sum5/2, Sum6/2
  Unit Delay2/1 -> Relational Operator3/2, Relational Operator1/2
  Relational Operator3/1 -> Sync -/1
  Relational Operator1/1 -> Sync +/1
  alpha2/1 -> Sum5/1, Sum6/1
  Sum5/1 -> Relational Operator/2
  Sum6/1 -> Relational Operator2/2
  Relational Operator/1 -> Logical Operator2/1
  Logical Operator2/1 -> Latch/1(S)
  Latch/2(0) -> Unit Delay/1
  Unit Delay/1 -> Logical Operator2/2
  Relational Operator2/1 -> Logical Operator4/1
  Logical Operator4/1 -> Latch/2(R)
  Unit Delay1/1 -> Logical Operator4/2
  Latch/1(1) -> Relational Operator3/1, Relational Operator1/1, Unit Delay2/1, Unit Delay1/1, SqWave/1
  Product2/1 -> Trigonometric Function7/1
  alpha9/1 -> Product2/1

== system MATLABPSB_BASED_MODELING_AND_Sim/SS2/SVC Controller/Firing Unit/Firing Unit BC/BL4 ==
  note: Note: Sync+ , Sync - and SqWave signals are inverted for TSC firing (i.e. positive thyristor is fired on negative peak voltage)
  SqWave : Inport  PortDimensions=1
  Sync + : Inport  Port=2  PortDimensions=1
  Sync - : Inport  Port=3  PortDimensions=1
  TSC_On : Inport  Port=4  PortDimensions=1
  Alpha1 : Constant  Value=FiringMode-1
  Logical Operator1 : Logic  Operator=NOT
  Logical Operator10 : Logic  Operator=OR
  Logical Operator11 : Logic  Inputs=3
  Logical Operator12 : Logic
  Logical Operator13 : Logic
  Logical Operator14 : Logic  Operator=OR
  Logical Operator15 : Logic  Inputs=3
  Switch5 : Switch  Threshold=0.5  SaturateOnIntegerOverflow=on  InputSameDT=on
  Switch6 : Switch  Threshold=0.5  SaturateOnIntegerOverflow=on  InputSameDT=on
  Transport Delay : TransportDelay  DelayTime=1/FreqInit  BufferSize=2048
  Unit Delay6 : UnitDelay  SampleTime=Ts
  Unit Delay7 : UnitDelay  SampleTime=Ts
  TSC + : Outport
  TSC - : Outport  Port=2
  wires:
  Unit Delay6/1 -> Switch5/3
  Unit Delay7/1 -> Switch6/3
  Sync +/1 -> Switch6/2
  Sync -/1 -> Switch5/2
  TSC_On/1 -> Switch5/1, Switch6/1, Logical Operator11/3, Logical Operator15/3
  Logical Operator13/1 -> Logical Operator12/1
  Alpha1/1 -> Logical Operator12/2
  Logical Operator12/1 -> Transport Delay/1
  SqWave/1 -> Logical Operator1/1, Logical Operator14/1
  Switch5/1 -> Unit Delay6/1, Logical Operator13/1, Logical Operator11/1
  Switch6/1 -> Unit Delay7/1, Logical Operator13/2, Logical Operator15/1
  Logical Operator1/1 -> Logical Operator10/1
  Logical Operator10/1 -> Logical Operator11/2
  Logical Operator14/1 -> Logical Operator15/2
  Logical Operator11/1 -> TSC +/1
  Logical Operator15/1 -> TSC -/1
  Transport Delay/1 -> Logical Operator10/2, Logical Operator14/2

== system MATLABPSB_BASED_MODELING_AND_Sim/SS2/SVC Controller/Firing Unit/Firing Unit BC/BL5 ==
  note: Note: Sync+ , Sync - and SqWave signals are inverted for TSC firing (i.e. positive thyristor is fired on negative peak voltage)
  SqWave : Inport  PortDimensions=1
  Sync + : Inport  Port=2  PortDimensions=1
  Sync - : Inport  Port=3  PortDimensions=1
  TSC_On : Inport  Port=4  PortDimensions=1
  Alpha1 : Constant  Value=FiringMode-1
  Logical Operator1 : Logic  Operator=NOT
  Logical Operator10 : Logic  Operator=OR
  Logical Operator11 : Logic  Inputs=3
  Logical Operator12 : Logic
  Logical Operator13 : Logic
  Logical Operator14 : Logic  Operator=OR
  Logical Operator15 : Logic  Inputs=3
  Switch5 : Switch  Threshold=0.5  SaturateOnIntegerOverflow=on  InputSameDT=on
  Switch6 : Switch  Threshold=0.5  SaturateOnIntegerOverflow=on  InputSameDT=on
  Transport Delay : TransportDelay  DelayTime=1/FreqInit  BufferSize=2048
  Unit Delay6 : UnitDelay  SampleTime=Ts
  Unit Delay7 : UnitDelay  SampleTime=Ts
  TSC + : Outport
  TSC - : Outport  Port=2
  wires:
  Transport Delay/1 -> Logical Operator14/2, Logical Operator10/2
  Logical Operator15/1 -> TSC -/1
  Logical Operator11/1 -> TSC +/1
  Logical Operator14/1 -> Logical Operator15/2
  Logical Operator10/1 -> Logical Operator11/2
  Logical Operator1/1 -> Logical Operator10/1
  Switch6/1 -> Logical Operator15/1, Logical Operator13/2, Unit Delay7/1
  Switch5/1 -> Logical Operator11/1, Logical Operator13/1, Unit Delay6/1
  SqWave/1 -> Logical Operator14/1, Logical Operator1/1
  Logical Operator12/1 -> Transport Delay/1
  Alpha1/1 -> Logical Operator12/2
  Logical Operator13/1 -> Logical Operator12/1
  TSC_On/1 -> Logical Operator15/3, Logical Operator11/3, Switch6/1, Switch5/1
  Sync -/1 -> Switch5/2
  Sync +/1 -> Switch6/2
  Unit Delay7/1 -> Switch6/3
  Unit Delay6/1 -> Switch5/3

== system MATLABPSB_BASED_MODELING_AND_Sim/SS2/SVC Controller/Firing Unit/Firing Unit BC/BL6 ==
  note: Note: Sync+ , Sync - and SqWave signals are inverted for TSC firing (i.e. positive thyristor is fired on negative peak voltage)
  SqWave : Inport  PortDimensions=1
  Sync + : Inport  Port=2  PortDimensions=1
  Sync - : Inport  Port=3  PortDimensions=1
  TSC_On : Inport  Port=4  PortDimensions=1
  Alpha1 : Constant  Value=FiringMode-1
  Logical Operator1 : Logic  Operator=NOT
  Logical Operator10 : Logic  Operator=OR
  Logical Operator11 : Logic  Inputs=3
  Logical Operator12 : Logic
  Logical Operator13 : Logic
  Logical Operator14 : Logic  Operator=OR
  Logical Operator15 : Logic  Inputs=3
  Switch5 : Switch  Threshold=0.5  SaturateOnIntegerOverflow=on  InputSameDT=on
  Switch6 : Switch  Threshold=0.5  SaturateOnIntegerOverflow=on  InputSameDT=on
  Transport Delay : TransportDelay  DelayTime=1/FreqInit  BufferSize=2048
  Unit Delay6 : UnitDelay  SampleTime=Ts
  Unit Delay7 : UnitDelay  SampleTime=Ts
  TSC + : Outport
  TSC - : Outport  Port=2
  wires:
  Unit Delay6/1 -> Switch5/3
  Unit Delay7/1 -> Switch6/3
  Sync +/1 -> Switch6/2
  Sync -/1 -> Switch5/2
  TSC_On/1 -> Switch5/1, Switch6/1, Logical Operator11/3, Logical Operator15/3
  Logical Operator13/1 -> Logical Operator12/1
  Alpha1/1 -> Logical Operator12/2
  Logical Operator12/1 -> Transport Delay/1
  SqWave/1 -> Logical Operator1/1, Logical Operator14/1
  Switch5/1 -> Unit Delay6/1, Logical Operator13/1, Logical Operator11/1
  Switch6/1 -> Unit Delay7/1, Logical Operator13/2, Logical Operator15/1
  Logical Operator1/1 -> Logical Operator10/1
  Logical Operator10/1 -> Logical Operator11/2
  Logical Operator14/1 -> Logical Operator15/2
  Logical Operator11/1 -> TSC +/1
  Logical Operator15/1 -> TSC -/1
  Transport Delay/1 -> Logical Operator10/2, Logical Operator14/2
